simulink model "TestBench_DSD"  (R2021a)
settings: Solver=VariableStepAuto  StartTime=0.0  StopTime=0.05  FixedStep=1e-10  MaxStep=1e-4  RelTol=1e-3
PreLoadFcn:
  | clear;
  | dead_time= 5e-7;
  | T_sample = 1e-7;
  | f_pwm= 8e3;
  | f_el=200;
  | amplitude=0.1;
  | U_dc=800;
  | Iq_soll=200;
  | 
  | load('busdef.mat')
  | 
  | %**** Controller ****
  | L_filter = 70e-6;
  | R_losses = 1.74e-3;
  | PGain = L_filter*0.05*2*pi;
  | IGain = R_losses*0.05*2*pi;
  | 
  | %**** Deadtime Correction ****
  | Rds_on_module = 0.045/15;
  | 
  | %**** Filter ****
  | FilterQuality = 0.7071
InitFcn:
  | %%PGain = (L_filter*0.09*2*pi*f_pwm-R_losses)*0.45;
  | %%IGain = PGain*50/1.2; %% 25 = Period for ringing with too hight PGain
  | 
  | %%PGain = L_filter/(2*(1.5/f_pwm));
  | %%IGain  = PGain*R_losses/L_filter;
undefined symbols (not defined in the file): DiscIntNeverNeededParam, haltPwmSi, haltPwmSic, I_abc_sampled
libraries: nesl_utility x18, simulink x17, fl_lib x15, ee_lib x5, spsFirstOrderFilterLib x3, eeTransforms x2, cstextras x1, spsRMSLib x1, simulink_extras x1, spspowerguiLib x1
(part 3 of 3)

== matlab function TestBench_DSD/Controller/Function-Call Subsystem8/MATLAB Function ==
  data: phase input; y output Bus: Device; devBus input Bus: Device
function y = fcn(phase,devBus)

switch phase 

    case 1

        devBus.U.Sic.ChB.TOn.enable = inf;
        devBus.U.Si.ChB.TOn.enable  = 1;

    case 2

        devBus.V.Sic.ChB.TOn.enable = inf;
        devBus.V.Si.ChB.TOn.enable  = 1;

    case 3

        devBus.W.Sic.ChB.TOn.enable = inf;
        devBus.W.Si.ChB.TOn.enable  = 1;
    
    otherwise
        error('No phase specified');

end

y = devBus;
